simulink model "p"  (Simulink 2.09)
settings: Solver=ode45  StartTime=0.0  StopTime=5700*2  RelTol=1e-3  AbsTol=1e-3
values from neighbouring files (symbols this model uses):
  w = 7    [Apid_hf1.m]    (also in alapjel.m = 7.5; e.m = be(1); picont.m = be(1))
libraries: simulink x1
settings Model: SaveTime=off  SaveOutput=off  ConsistencyChecking=off  RTWTemplateMakefile=grt_vc.tmf

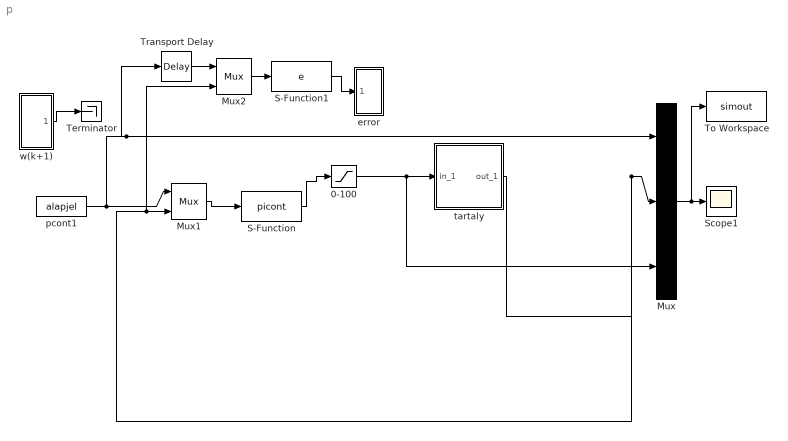
== system p ==
  0-100 : Saturate  UpperLimit=100  LowerLimit=0
  Mux : Mux  Inputs=3
  Mux1 : Mux  Inputs=2
  Mux2 : Mux  Inputs=2
  S-Function : S-Function  FunctionName=picont
  S-Function1 : S-Function  FunctionName=e
  Scope1 : Scope
      settings: TickLabels=on  TimeRange=5700  YMin=0  YMax=80  SaveName=pi  SampleInput=on
  Terminator : Terminator
  To Workspace : ToWorkspace  VariableName=simout  SampleTime=10
  Transport Delay : TransportDelay  DelayTime=10  InitialInput=w  BufferSize=1024
  error : Subsystem
      mask Display: disp('IAE')
  pcont1 : S-Function  FunctionName=alapjel
  tartaly : Subsystem
      mask Display: disp('Obj')
  w(k+1) : Subsystem
  wires:
  Mux/1 -> To Workspace/1, Scope1/1
  Transport Delay/1 -> Mux2/1
  Mux2/1 -> S-Function1/1
  S-Function1/1 -> error/1(in_1)
  S-Function/1 -> 0-100/1
  w(k+1)/1(out_1) -> Terminator/1
  pcont1/1 -> Transport Delay/1, Mux/1, Mux1/1
  tartaly/1(out_1) -> Mux2/2, Mux1/2, Mux/2
  0-100/1 -> tartaly/1(in_1), Mux/3
  Mux1/1 -> S-Function/1

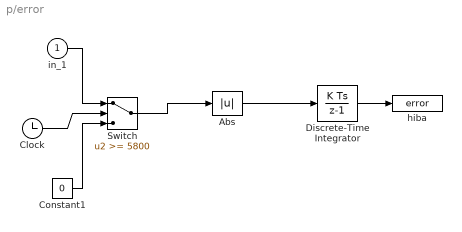
== system p/error ==
  in_1 : Inport  Port=1  PortWidth=-1  SampleTime=-1
  Abs : Abs
  Clock : Clock
  Constant1 : Constant  Value=0
  Discrete-Time Integrator : DiscreteIntegrator  IntegratorMethod=ForwardEuler  ExternalReset=none  InitialConditionSource=internal  InitialCondition=0  LimitOutput=off  UpperSaturationLimit=inf  LowerSaturationLimit=-inf  ShowSaturationPort=off  ShowStatePort=off  SampleTime=10
  Switch : Switch  Threshold=5800
  hiba : ToWorkspace  VariableName=error  SampleTime=0
      settings: Buffer=1
  wires:
  Switch/1 -> Abs/1
  in_1/1 -> Switch/1
  Constant1/1 -> Switch/3
  Clock/1 -> Switch/2
  Abs/1 -> Discrete-Time Integrator/1
  Discrete-Time Integrator/1 -> hiba/1

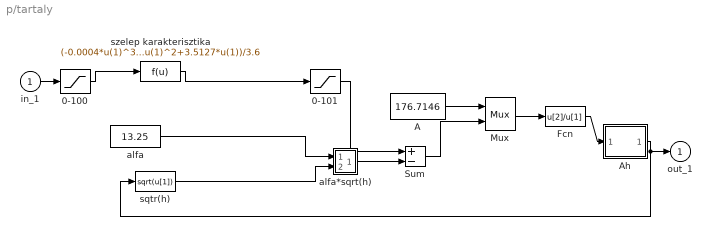
== system p/tartaly ==
  in_1 : Inport  Port=1  PortWidth=-1  SampleTime=-1
  0-100 : Saturate  UpperLimit=100  LowerLimit=0
  0-101 : Saturate  UpperLimit=140  LowerLimit=0
  A : Constant  Value=176.7146
  Ah : Subsystem  mask(Limited Integrator.){@1=2, @2=85, @3=w}
      mask prompts: @1 "Lower bound:"; @2 "Upper bound:"; @3 "Initial condition:"
      mask help: Limited Integrator
      mask init:
      | lower_limit=@1;upper_limit=@2;X0=@3;
      mask Help: Implements a limited integrator with \nan expression of the form:\n\nif(x<=lb and u<0) or (x>=ub and u>0)\n   xdot=0\nelse\n   xdot=u
      mask Display: plot(-1,-0.2,3.5,1.2,[0.05,1,2,2.9],[0,0,1,1]);disp(' 1/s    ')
  Fcn : Fcn  Expr=u[2]/u[1]
  Mux : Mux  Inputs=2
  Sum : Sum  Inputs=+-
  alfa : Constant  Value=13.25
  alfa*sqrt(h) : Subsystem
      mask Type: Dot Product
      mask Description:
      | Inner (dot) product.
      | y=sum(u1.*u2)
      mask Help: Computes the inner (dot) product of the inputs: sum(u1.*u2).  The inputs are vectors of the same length. Output is a scalar.
      mask Display: disp('.\n')
  sqtr(h) : Fcn  Expr=sqrt(u[1])
  szelep karakterisztika : Fcn  Expr=(-0.0004*u(1)^3+0.0571*u(1)^2+3.5127*u(1))/3.6
  out_1 : Outport  Port=1  InitialOutput=0
  wires:
  szelep karakterisztika/1 -> 0-101/1
  0-100/1 -> szelep karakterisztika/1
  in_1/1 -> 0-100/1
  alfa*sqrt(h)/1(out_1) -> Sum/2
  sqtr(h)/1 -> alfa*sqrt(h)/2(in_2)
  alfa/1 -> alfa*sqrt(h)/1(in_1)
  Mux/1 -> Fcn/1
  A/1 -> Mux/1
  Sum/1 -> Mux/2
  Fcn/1 -> Ah/1(Inport)
  Ah/1(Outport) -> out_1/1, sqtr(h)/1
  0-101/1 -> Sum/1

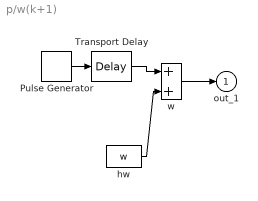
== system p/w(k+1) ==
  Pulse Generator : simulink/Sources/Pulse Generator  period=400  duty=50  amplitude=5  start=100
  Transport Delay : TransportDelay  DelayTime=200  InitialInput=0  BufferSize=1024
  hw : Constant  Value=w
  w : Sum  Inputs=++
  out_1 : Outport  Port=1  InitialOutput=0
  wires:
  w/1 -> out_1/1
  hw/1 -> w/2
  Pulse Generator/1 -> Transport Delay/1
  Transport Delay/1 -> w/1

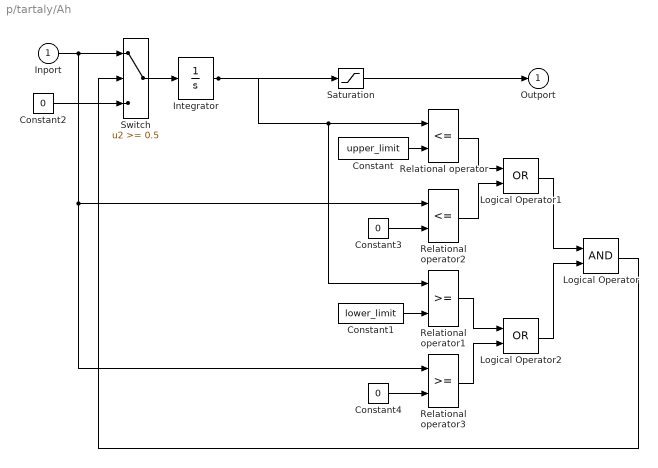
== system p/tartaly/Ah ==
  Inport : Inport  Port=1  PortWidth=-1  SampleTime=-1
  Constant : Constant  Value=upper_limit
  Constant1 : Constant  Value=lower_limit
  Constant2 : Constant  Value=0
  Constant3 : Constant  Value=0
  Constant4 : Constant  Value=0
  Integrator : Integrator  ExternalReset=none  InitialConditionSource=internal  InitialCondition=X0  LimitOutput=off  UpperSaturationLimit=inf  LowerSaturationLimit=-inf  ShowSaturationPort=off  ShowStatePort=off  AbsoluteTolerance=auto
  Logical Operator : Logic  Operator=AND  Inputs=2
  Logical Operator1 : Logic  Operator=OR  Inputs=2
  Logical Operator2 : Logic  Operator=OR  Inputs=2
  Relational operator : RelationalOperator  Operator=<=
  Relational operator1 : RelationalOperator  Operator=>=
  Relational operator2 : RelationalOperator  Operator=<=
  Relational operator3 : RelationalOperator  Operator=>=
  Saturation : Saturate  UpperLimit=upper_limit  LowerLimit=lower_limit
  Switch : Switch  Threshold=0.5
  Outport : Outport  Port=1  InitialOutput=0
  wires:
  Saturation/1 -> Outport/1
  Inport/1 -> Switch/1, Relational operator2/1, Relational operator3/1
  Switch/1 -> Integrator/1
  Constant/1 -> Relational operator/2
  Constant1/1 -> Relational operator1/2
  Logical Operator/1 -> Switch/2
  Constant2/1 -> Switch/3
  Relational operator/1 -> Logical Operator1/1
  Relational operator2/1 -> Logical Operator1/2
  Logical Operator1/1 -> Logical Operator/1
  Relational operator1/1 -> Logical Operator2/1
  Relational operator3/1 -> Logical Operator2/2
  Logical Operator2/1 -> Logical Operator/2
  Constant3/1 -> Relational operator2/2
  Constant4/1 -> Relational operator3/2
  Integrator/1 -> Saturation/1, Relational operator1/1, Relational operator/1

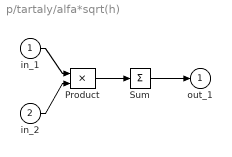
== system p/tartaly/alfa*sqrt(h) ==
  in_1 : Inport  Port=1  PortWidth=-1  SampleTime=-1
  in_2 : Inport  Port=2  PortWidth=-1  SampleTime=-1
  Product : Product  Inputs=2
  Sum : Sum  Inputs=+
  out_1 : Outport  Port=1  InitialOutput=0
  wires:
  in_2/1 -> Product/2
  in_1/1 -> Product/1
  Product/1 -> Sum/1
  Sum/1 -> out_1/1
